simulink model "chap10_3sim"  (Simulink 3.00)
settings: Solver=ode45  StartTime=0.0  StopTime=10.0  RelTol=1e-3
settings Model: LastModifiedBy=liu

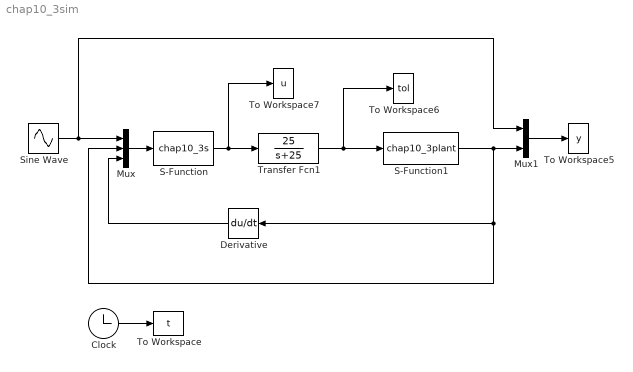
== system chap10_3sim ==
  Clock : Clock
  Derivative : Derivative  Orientation=left
  Mux : Mux  Inputs=3
  Mux1 : Mux  Inputs=2
  S-Function : S-Function  FunctionName=chap10_3s  PortCounts=[]  SFunctionModules=''
  S-Function1 : S-Function  FunctionName=chap10_3plant  PortCounts=[]  SFunctionModules=''
  Sine Wave : Sin  Amplitude=1  Frequency=2*pi  Phase=0  SampleTime=0
  To Workspace : ToWorkspace  VariableName=t  SampleTime=-1  SaveFormat=Matrix
  To Workspace5 : ToWorkspace  VariableName=y  SampleTime=-1  SaveFormat=Matrix
  To Workspace6 : ToWorkspace  VariableName=tol  SampleTime=-1  SaveFormat=Matrix
  To Workspace7 : ToWorkspace  VariableName=u  SampleTime=-1  SaveFormat=Matrix
  Transfer Fcn1 : TransferFcn  Numerator=[25]  Denominator=[1 25]
  wires:
  Mux/1 -> S-Function/1
  Derivative/1 -> Mux/3
  Sine Wave/1 -> Mux/1, Mux1/1
  Mux1/1 -> To Workspace5/1
  S-Function1/1 -> Derivative/1, Mux/2, Mux1/2
  S-Function/1 -> To Workspace7/1, Transfer Fcn1/1
  Clock/1 -> To Workspace/1
  Transfer Fcn1/1 -> S-Function1/1, To Workspace6/1
